simulink model "a"  (R2021b)
settings: Solver=VariableStepAuto  StartTime=0.0  StopTime=18  MinStep=0.0001  RelTol=1e-3
settings Model: Creator=linggm  LastModifiedBy=linggm

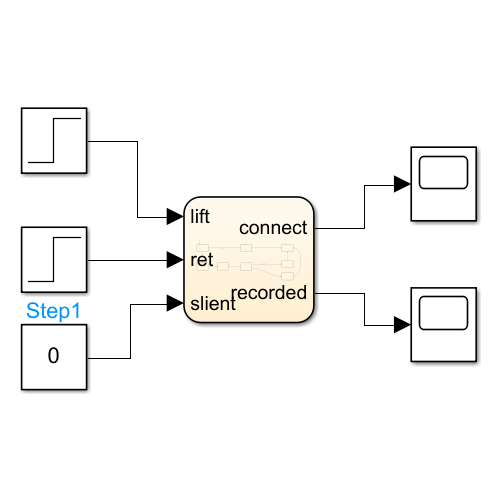
[thumbnail: Simulink's stored preview of the top-level diagram]
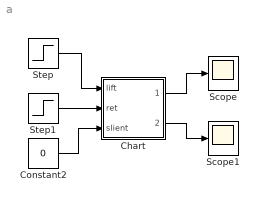
== system a ==
  Chart : Stateflow chart  TreatAsAtomicUnit=on
  Constant2 : Constant  Value=0
  Scope : Scope
  Scope1 : Scope
  Step : Step  Time=2  SampleTime=0
  Step1 : Step  Time=6  SampleTime=0
  wires:
  Step/1 -> Chart/1(lift)
  Chart/1(connect) -> Scope/1
  Step1/1 -> Chart/2(ret)
  Constant2/1 -> Chart/3(slient)
  Chart/2(recorded) -> Scope1/1

== stateflow chart a/Chart ==
  state ring
    connect=0;
  state dead
    connect=0;
  state talk
    connect=1;
  state beep1
    connect=0;
    recorded=1;
  state play_text
    connect=0;
  state beep
    connect=0;
  state record
    connect=0;
  state beep2
    connect=0;
    recorded=0;
  (default) -> ring
  beep2 -> dead
  ring -> (junction 21) [order 1] : [lift ==  1]
  (junction 21) -> talk : [before(4, sec)]
  talk -> dead : [ret==1]
  ring -> play_text [order 2] : [after(4, sec)]
  beep1 -> dead
  record -> (junction 49) [order 1] : [slient == 0]
  (junction 49) -> beep1 : [after(8, sec)]
  play_text -> beep
  beep -> record
  record -> beep2 [order 2] : [slient == 1]
  data: lift input; ret input; slient input; connect output; recorded output
